simulink model "HybridSimulator"  (Simulink 7.6)
settings: Solver=ode23  StartTime=0.0  StopTime=T  MaxStep=0.001  RelTol=1e-8
values from neighbouring files (symbols this model uses):
  J = j(length(j))    [plotHybridArc.m]    (also in plotflows.m; plotjumps.m; run.m = 20)
  rule = 1    [run.m]
  T = t(length(t))    [plotHybridArc.m]    (also in plotflows.m; plotjumps.m; run.m = 10)
  x0 = [5;0]    [run.m]
  z0 = [x0; u0]    [run.m]
undefined symbols (not defined in the file or in its folder): C, D, f, g, jumpPriority, O
libraries: simulink x2
settings Model: Creator=rsanfelice  LastModifiedBy=dacopp  ExtModeAutoUpdateStatusClock=off
settings OptimizationCC: BlockReduction=off  BooleanDataType=off  InitFltsAndDblsToZero=on
settings DebuggingCC: AlgebraicLoopMsg=none  SaveWithParameterizedLinksMsg=none  SignalResolutionControl=TryResolveAllWithWarning  SolverPrmCheckMsg=none  MultiTaskDSMMsg=warning  MultiTaskCondExecSysMsg=none  StrictBusMsg=None
settings HardwareCC: TargetUnknown=on
settings RTWCC: IncludeERTFirstTime=on
settings GRTTargetCC: TargetFcnLib=ansi_tfl_tmw.mat

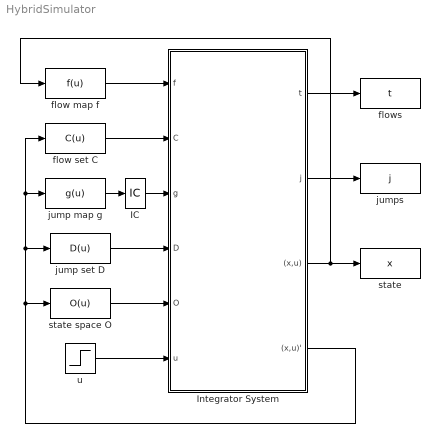
== system HybridSimulator ==
  IC : InitialCondition  Value=x0
  Integrator System : Subsystem
  flow map f : MATLABFcn  MATLABFcn=f(u)
  flow set C : MATLABFcn  MATLABFcn=C(u)
  flows : ToWorkspace  VariableName=t  SampleTime=-1  SaveFormat=Array
  jump map g : MATLABFcn  MATLABFcn=g(u)
  jump set D : MATLABFcn  MATLABFcn=D(u)
  jumps : ToWorkspace  VariableName=j  SampleTime=-1  SaveFormat=Array
  state : ToWorkspace  VariableName=x  SampleTime=-1  SaveFormat=Array
  state space O : MATLABFcn  MATLABFcn=O(u)
  u : Step  Time=0  After=.2  SampleTime=0
  wires:
  jump map g/1 -> IC/1
  jump set D/1 -> Integrator System/4(D)
  flow map f/1 -> Integrator System/1(f)
  Integrator System/4((x,u)') -> jump set D/1, jump map g/1, flow set C/1, state space O/1
  IC/1 -> Integrator System/3(g)
  Integrator System/3((x,u)) -> state/1, flow map f/1
  flow set C/1 -> Integrator System/2(C)
  Integrator System/1(t) -> flows/1
  Integrator System/2(j) -> jumps/1
  state space O/1 -> Integrator System/5(O)
  u/1 -> Integrator System/6(u)

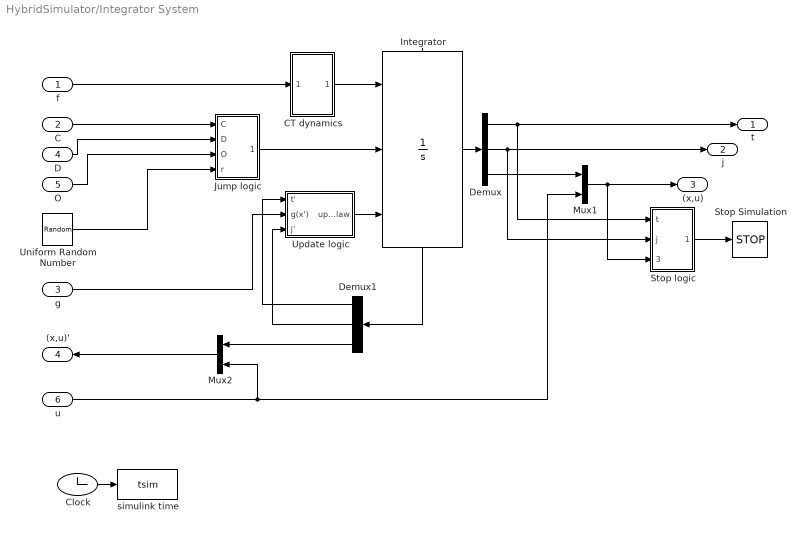
== system HybridSimulator/Integrator System ==
  f : Inport
  C : Inport  Port=2
  g : Inport  Port=3
  D : Inport  Port=4
  O : Inport  Port=5
  u : Inport  Port=6
  CT dynamics : Subsystem
  Clock : Clock
      settings: Decimation=10
  Demux : Demux  Outputs=[1 1 -1]
  Demux1 : Demux  Outputs=[1 1 -1]
  Integrator : Integrator  ExternalReset=level hold  InitialConditionSource=external  ShowStatePort=on  ZeroCross=off
  Jump logic : Subsystem
  Mux1 : Mux  Inputs=2
  Mux2 : Mux  Inputs=2
  Stop Simulation : Stop
  Stop logic : Subsystem
  Uniform Random Number : UniformRandomNumber  Minimum=0  Seed=abs(floor(100*rand))  SampleTime=0
  Update logic : Subsystem
  simulink time : ToWorkspace  VariableName=tsim  SampleTime=-1  SaveFormat=Array
  t : Outport
  j : Outport  Port=2
  (x,u) : Outport  Port=3
  (x,u)' : Outport  Port=4
  wires:
  Demux/2 -> j/1, Stop logic/2(j)
  Demux/1 -> t/1, Stop logic/1(t)
  Demux1/2 -> Update logic/3(j')
  Demux1/1 -> Update logic/1(t')
  Update logic/1(update law) -> Integrator/3
  Integrator/State -> Demux1/1
  CT dynamics/1(dot) -> Integrator/1
  Stop logic/1(stop) -> Stop Simulation/1
  Integrator/1 -> Demux/1
  C/1 -> Jump logic/1(C)
  D/1 -> Jump logic/2(D)
  O/1 -> Jump logic/3(O)
  f/1 -> CT dynamics/1(f(x))
  Demux1/3 -> Mux2/1
  Clock/1 -> simulink time/1
  g/1 -> Update logic/2(g(x'))
  Jump logic/1(jump) -> Integrator/2
  Uniform Random Number/1 -> Jump logic/4(r)
  Demux/3 -> Mux1/1
  Mux1/1 -> (x,u)/1, Stop logic/3((x,u))
  u/1 -> Mux2/2, Mux1/2
  Mux2/1 -> (x,u)'/1

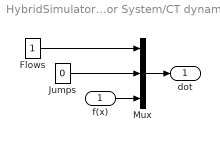
== system HybridSimulator/Integrator System/CT dynamics ==
  f(x) : Inport
  Flows : Constant
  Jumps : Constant  Value=0
  Mux : Mux  Inputs=[1 1 -1]
  dot : Outport
  wires:
  Jumps/1 -> Mux/2
  Flows/1 -> Mux/1
  Mux/1 -> dot/1
  f(x)/1 -> Mux/3

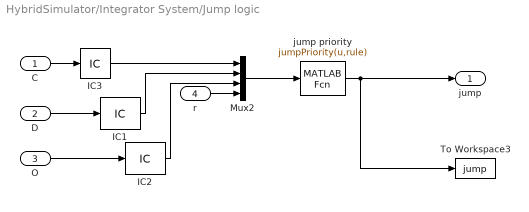
== system HybridSimulator/Integrator System/Jump logic ==
  C : Inport
  D : Inport  Port=2
  O : Inport  Port=3
  r : Inport  Port=4
  IC1 : InitialCondition  Value=D(z0)
  IC2 : InitialCondition  Value=O(z0)
  IC3 : InitialCondition  Value=C(z0)
  Mux2 : Mux
  To Workspace3 : ToWorkspace  VariableName=jump  SampleTime=-1  SaveFormat=Array
  jump priority : MATLABFcn  MATLABFcn=jumpPriority(u,rule)
  jump : Outport
  wires:
  IC3/1 -> Mux2/1
  IC1/1 -> Mux2/2
  Mux2/1 -> jump priority/1
  jump priority/1 -> jump/1, To Workspace3/1
  IC2/1 -> Mux2/3
  C/1 -> IC3/1
  r/1 -> Mux2/4
  D/1 -> IC1/1
  O/1 -> IC2/1

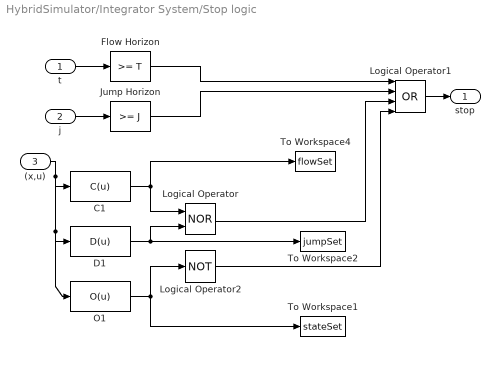
== system HybridSimulator/Integrator System/Stop logic ==
  t : Inport
  j : Inport  Port=2
  (x,u) : Inport  Port=3
  C1 : MATLABFcn  MATLABFcn=C(u)
  D1 : MATLABFcn  MATLABFcn=D(u)
  Flow Horizon : simulink/Logic and Bit Operations/Compare To Constant  SystemSampleTime=-1  relop=>=  const=T  LogicOutDataTypeMode=uint8  ZeroCross=off
  Jump Horizon : simulink/Logic and Bit Operations/Compare To Constant  SystemSampleTime=-1  relop=>=  const=J  LogicOutDataTypeMode=uint8  ZeroCross=off
  Logical Operator : Logic  Operator=NOR  AllPortsSameDT=off  OutDataTypeStr=boolean
  Logical Operator1 : Logic  Operator=OR  Inputs=4  AllPortsSameDT=off  OutDataTypeStr=boolean
  Logical Operator2 : Logic  Operator=NOT  AllPortsSameDT=off  OutDataTypeStr=boolean
  O1 : MATLABFcn  MATLABFcn=O(u)
  To Workspace1 : ToWorkspace  VariableName=stateSet  SampleTime=-1  SaveFormat=Array
  To Workspace2 : ToWorkspace  VariableName=jumpSet  SampleTime=-1  SaveFormat=Array
  To Workspace4 : ToWorkspace  VariableName=flowSet  SampleTime=-1  SaveFormat=Array
  stop : Outport
  wires:
  Flow Horizon/1 -> Logical Operator1/1
  Jump Horizon/1 -> Logical Operator1/2
  Logical Operator/1 -> Logical Operator1/3
  C1/1 -> Logical Operator/1, To Workspace4/1
  Logical Operator2/1 -> Logical Operator1/4
  D1/1 -> Logical Operator/2, To Workspace2/1
  O1/1 -> Logical Operator2/1, To Workspace1/1
  t/1 -> Flow Horizon/1
  j/1 -> Jump Horizon/1
  (x,u)/1 -> C1/1, O1/1, D1/1
  Logical Operator1/1 -> stop/1

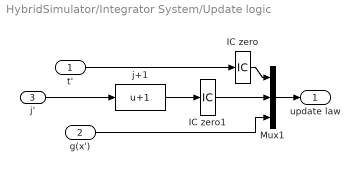
== system HybridSimulator/Integrator System/Update logic ==
  t' : Inport
  g(x') : Inport  Port=2
  j' : Inport  Port=3
  IC zero : InitialCondition  Value=0
  IC zero1 : InitialCondition  Value=0
  Mux1 : Mux  Inputs=[1 1 -1]
  j+1 : MATLABFcn  MATLABFcn=u+1
  update law : Outport
  wires:
  IC zero1/1 -> Mux1/2
  j+1/1 -> IC zero1/1
  IC zero/1 -> Mux1/1
  t'/1 -> IC zero/1
  Mux1/1 -> update law/1
  j'/1 -> j+1/1
  g(x')/1 -> Mux1/3
